simulink model "exp2"  (R2018a)
settings: Solver=VariableStepAuto  StartTime=0.0  StopTime=10.0  RelTol=1e-3
undefined symbols (not defined in the file): Ion, Lithium
libraries: powerlib x5, electricdrivelib x1
settings Model: Creator=Bhaskar  LastModifiedBy=Bhaskar

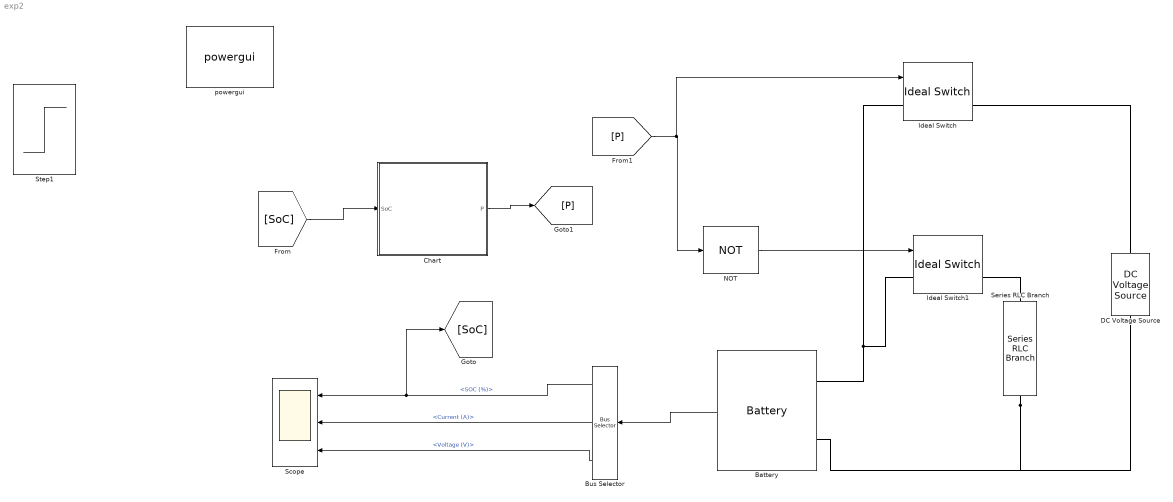
== system exp2 ==
  Battery : electricdrivelib/Extra Sources/Battery  BatType=Lithium-Ion  ShowTempParam=off  ThermalPreset=no  ShowAgeParam=off  NomV=7  NomQ=2  SOC=50  Batt_Tr=30  PresetModel=off  MaxQ=5.4  MinV=5.4  FullV=8.3807  Dis_rate=2.3478  R=0.013333  Normal_OP=4.8835  expZone="[7.7788      0.2653]"  current=[6.5 13 32.5]  Units=Time  Tci=20  NomT=20  T2=-30  MaxQ2=4.8  FullV2=7.1  Normal_OP2=5.655  expZone2="[6.58           1]"  Rca=0.6  ti=2000  Dp=0  Neq0=0  Tsim=1e6  Ta1=25  Qeol=5.4*0.9  Reol=0.013333*1.2  Char_age=[2.3478, 3]  Dis_age=[2.3478, 10]  N1=1500  N2=10500  N3=1000  N4=1400  Ta2=45  N5=950
  Bus Selector : BusSelector  OutputSignals=SOC (%),Current (A),Voltage (V)
  Chart : Stateflow chart  TreatAsAtomicUnit=on
  DC Voltage Source : powerlib/Electrical Sources/DC Voltage Source  Amplitude=7*1.1  Measurements=None
  Ideal Switch : powerlib/Power Electronics/Ideal Switch  Ron=0.001  Lon=0  IC=0  Rs=1e5  Cs=inf  Measurements=on
  Ideal Switch1 : powerlib/Power Electronics/Ideal Switch  Ron=0.001  Lon=0  IC=0  Rs=1e5  Cs=inf  Measurements=on
  NOT : Logic  Operator=NOT  IconShape=distinctive  AllPortsSameDT=off  OutDataTypeStr=boolean
  Scope : Scope  NumInputPorts=3
  Series RLC Branch : powerlib/Elements/Series RLC Branch  LConnTagsString=__new0  RConnTagsString=__new0  BranchType=R  Resistance=7/5  Inductance=1e-3  SetiL0=off  InitialCurrent=0  Capacitance=1e-6  Setx0=off  InitialVoltage=0  Measurements=None
  Step1 : Step  Time=5  SampleTime=0
  powergui : powerlib/powergui  Priority=1  SimulationMode=Continuous  SampleTime=50e-6  frequency=60  Iterations=50  frequencyindice=0  Pbase=100e6  ErrMax=1e-4  UnitsV=kV  UnitsW=MW  buscounter=0  FunctionMessages=off  echomessages=off  EnableUseOfTLC=off  CurrentSourceSwitches=off  DisableSnubberDevices=off  DisableRonSwitches=off  DisableVfSwitches=off  DisplayEquations=off  SolverType=Tustin/Backward Euler (TBE)  Interpol=off  ExternalGateDelay=off  methode=off  Ts=100  x0status=blocks  SPID=on  SwTol=0  HookPort=off  RestoreLinks=warning  ResistiveCurrentMeasurement=off  Frange=[0:2:500]  Ylog=off  Xlog=on  ShowGrid=off  save=off  variable=ZData  structure=0  ZoomFFT=off  StartTime=0.0  cycles=1  DisplayStyle=1  fundamental=60  FreqAxis=off  MaxFrequency=1000  frequencyindicesteady=1  RmsSteady=1  display=off
  wires:
  NOT/1 -> Ideal Switch1/1
  Battery/1 -> Bus Selector/1
  Bus Selector/2 -> Scope/2  "<Current (A)>"
  Bus Selector/1 -> [SoC], Scope/1  "<SOC (%)>"
  Bus Selector/3 -> Scope/3  "<Voltage (V)>"
  [P] -> Ideal Switch/1, NOT/1
  Chart/1(P) -> [P]
  [SoC] -> Chart/1(SoC)
  connections:
  Series RLC Branch/RConn1 -- Battery/LConn2 -- DC Voltage Source/LConn1
  DC Voltage Source/RConn1 -- Ideal Switch/RConn1
  Ideal Switch/LConn1 -- Battery/LConn1 -- Ideal Switch1/LConn1
  Ideal Switch1/RConn1 -- Series RLC Branch/LConn1

== stateflow chart exp2/Chart ==
  state Discharge [group]
    entry : P=0
  state Charge [group]
    entry : P=1
  (default) -> Discharge : [SoC>80]
  Discharge -> Charge : [SoC<20]
  data: P output; SoC input
